simulink model "exp_20230308_sistema_trifasico"  (R2022b)
settings: Solver=VariableStepAuto  StartTime=0.0  StopTime=10.0  RelTol=1e-3
undefined symbols (not defined in the file or in its folder): Angle, Magnitude
libraries: spsSeriesRLCBranchLib x7, spsCurrentMeasurementLib x4, spsACVoltageSourceLib x3, spsVoltageMeasurementLib x2, sps_lib x1
settings Model: Creator=miguel  LastModifiedBy=miguel

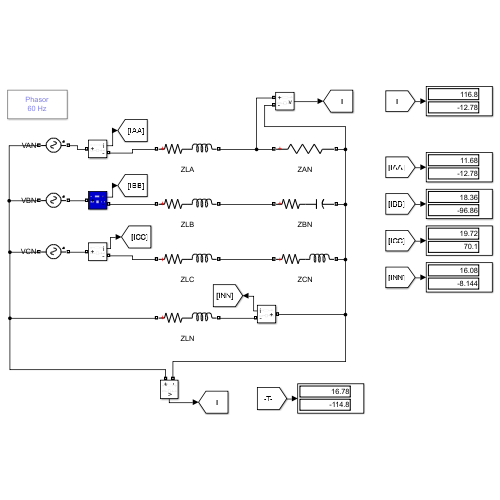
[thumbnail: Simulink's stored preview of the top-level diagram]
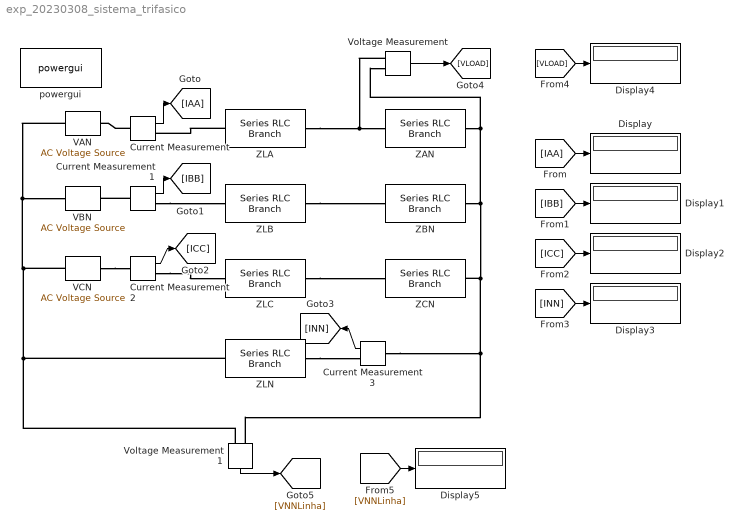
== system exp_20230308_sistema_trifasico ==
  Current Measurement{,1..3} (4 alike) : spsCurrentMeasurementLib/Current Measurement  PhasorSimulation=on  OutputType=Magnitude-Angle  PSBequivalent=0
  Display{,1..5} (6 alike) : Display
  VAN : spsACVoltageSourceLib/AC Voltage Source  Amplitude=127  Phase=0  Frequency=60  SampleTime=0  Measurements=None  BusType=swing  Pref=10e3  Qref=0  Qmin=-inf  Qmax=+inf
  VBN : spsACVoltageSourceLib/AC Voltage Source  Amplitude=127  Phase=-120  Frequency=60  SampleTime=0  Measurements=None  BusType=swing  Pref=10e3  Qref=0  Qmin=-inf  Qmax=+inf
  VCN : spsACVoltageSourceLib/AC Voltage Source  Amplitude=127  Phase=120  Frequency=60  SampleTime=0  Measurements=None  BusType=swing  Pref=10e3  Qref=0  Qmin=-inf  Qmax=+inf
  Voltage Measurement : spsVoltageMeasurementLib/Voltage Measurement  PhasorSimulation=on  OutputType=Magnitude-Angle  PSBequivalent=0
  Voltage Measurement1 : spsVoltageMeasurementLib/Voltage Measurement  PhasorSimulation=on  OutputType=Magnitude-Angle  PSBequivalent=0
  ZAN : spsSeriesRLCBranchLib/Series RLC Branch  LConnTagsString=__new0  RConnTagsString=__new0  BranchType=R  Resistance=10  Inductance=1/(2*pi*60)  SetiL0=off  InitialCurrent=0  Capacitance=1e-6  Setx0=off  InitialVoltage=0  Measurements=Branch voltage and current
  ZBN : spsSeriesRLCBranchLib/Series RLC Branch  LConnTagsString=__new0  RConnTagsString=__new0  BranchType=RC  Resistance=6.9282  Inductance=1/(2*pi*60)  SetiL0=off  InitialCurrent=0  Capacitance=1/(4*2*pi*60)  Setx0=off  InitialVoltage=0  Measurements=Branch voltage and current
  ZCN : spsSeriesRLCBranchLib/Series RLC Branch  LConnTagsString=__new0  RConnTagsString=__new0  BranchType=RL  Resistance=3  Inductance=4/(2*pi*60)  SetiL0=off  InitialCurrent=0  Capacitance=1e-6  Setx0=off  InitialVoltage=0  Measurements=Branch voltage and current
  ZLA : spsSeriesRLCBranchLib/Series RLC Branch  LConnTagsString=__new0  RConnTagsString=__new0  BranchType=RL  Resistance=0.3  Inductance=1/(2*pi*60)  SetiL0=off  InitialCurrent=0  Capacitance=1e-6  Setx0=off  InitialVoltage=0  Measurements=Branch voltage and current
  ZLB : spsSeriesRLCBranchLib/Series RLC Branch  LConnTagsString=__new0  RConnTagsString=__new0  BranchType=RL  Resistance=0.3  Inductance=1/(2*pi*60)  SetiL0=off  InitialCurrent=0  Capacitance=1e-6  Setx0=off  InitialVoltage=0  Measurements=None
  ZLC : spsSeriesRLCBranchLib/Series RLC Branch  LConnTagsString=__new0  RConnTagsString=__new0  BranchType=RL  Resistance=0.3  Inductance=1/(2*pi*60)  SetiL0=off  InitialCurrent=0  Capacitance=1e-6  Setx0=off  InitialVoltage=0  Measurements=None
  ZLN : spsSeriesRLCBranchLib/Series RLC Branch  LConnTagsString=__new0  RConnTagsString=__new0  BranchType=RL  Resistance=0.3  Inductance=1/(2*pi*60)  SetiL0=off  InitialCurrent=0  Capacitance=1e-6  Setx0=off  InitialVoltage=0  Measurements=None
  powergui : sps_lib/powergui  Priority=1  SimulationMode=Phasor  SampleTime=50e-6  frequency=60  Iterations=50  frequencyindice=60  Pbase=100e6  ErrMax=1e-4  UnitsV=kV  UnitsW=MW  buscounter=0  FunctionMessages=off  echomessages=off  EnableUseOfTLC=off  CurrentSourceSwitches=off  DisableSnubberDevices=off  DisableRonSwitches=off  DisableVfSwitches=off  DisplayEquations=off  AutomaticDiscreteSolvers=off  SolverType=Tustin/Backward Euler (TBE)  Interpol=off  ExternalGateDelay=off  methode=off  Ts=100  x0status=blocks  SPID=on  SwTol=0  HookPort=off  NonlinearTolerance=1e-4  nMaxIteration=100  ContinueOnMaxIteration=off  RestoreLinks=warning  ResistiveCurrentMeasurement=off  Frange=[0:2:500]  Ylog=off  Xlog=on  ShowGrid=off  save=off  variable=ZData  structure=0  ZoomFFT=off  StartTime=0.0  cycles=1  DisplayStyle=1  fundamental=60  FreqAxis=off  MaxFrequency=1000  frequencyindicesteady=1  RmsSteady=1  display=off
  wires:
  Current Measurement/1 -> [IAA]
  Current Measurement1/1 -> [IBB]
  Current Measurement2/1 -> [ICC]
  Current Measurement3/1 -> [INN]
  [IAA] -> Display/1
  [IBB] -> Display1/1
  [ICC] -> Display2/1
  [INN] -> Display3/1
  Voltage Measurement/1 -> [VLOAD]
  [VLOAD] -> Display4/1
  Voltage Measurement1/1 -> [VNNLinha]
  [VNNLinha] -> Display5/1
  connections:
  VCN/LConn1 -- Voltage Measurement1/LConn1 -- ZLN/LConn1 -- VAN/LConn1 -- VBN/LConn1
  Current Measurement/LConn1 -- VAN/RConn1
  ZLA/LConn1 -- Current Measurement/RConn1
  Current Measurement1/LConn1 -- VBN/RConn1
  VCN/RConn1 -- Current Measurement2/LConn1
  Current Measurement2/RConn1 -- ZLC/LConn1
  Current Measurement1/RConn1 -- ZLB/LConn1
  ZLA/RConn1 -- Voltage Measurement/LConn1 -- ZAN/LConn1
  ZLB/RConn1 -- ZBN/LConn1
  ZLC/RConn1 -- ZCN/LConn1
  Current Measurement3/LConn1 -- Voltage Measurement1/LConn2 -- ZAN/RConn1 -- Voltage Measurement/LConn2 -- ZBN/RConn1 -- ZCN/RConn1
  ZLN/RConn1 -- Current Measurement3/RConn1
